simulink model "HW_StateFeedback"  (R2026a)
settings: Solver=ode1  StopTime=30  FixedStep=0.002
undefined symbols (not defined in the file): HIL, K_aug_hw, K_E_SW, K_ec, K_gs, V_sat
libraries: quarc_library x4, seesaw_hw_lib x2
settings Model: Creator=Karim Negm  LastModifiedBy=Karim Negm

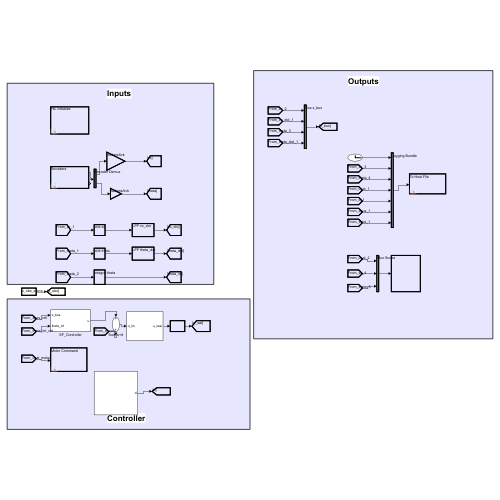
[thumbnail: Simulink's stored preview of the top-level diagram]
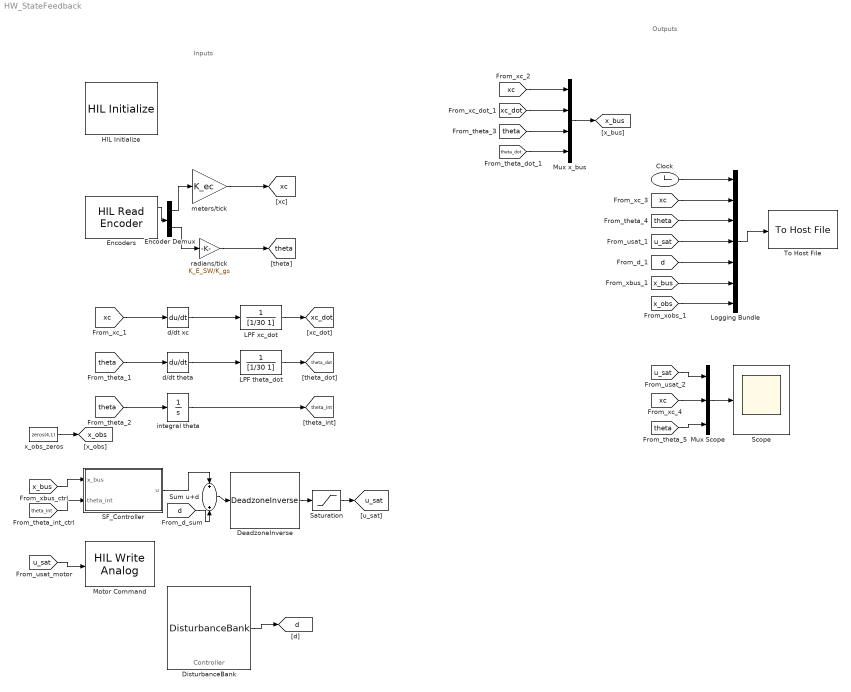
== system HW_StateFeedback ==
  note: Inputs
  note: Controller
  note: Outputs
  Clock : Clock
  DeadzoneInverse : seesaw_hw_lib/DeadzoneInverse  SystemSampleTime=-1  VariantActivationTime=update diagram  EmptyChoice=off  PassThrough=off  PassThroughVariantControl=(default)  EmptyChoiceVariantControl=(default)  AllowFlexibleInterface=on  Latency=0  AutoFrameSizeCalculation=off
  DisturbanceBank : seesaw_hw_lib/DisturbanceBank  SystemSampleTime=-1  VariantActivationTime=update diagram  EmptyChoice=off  PassThrough=off  PassThroughVariantControl=(default)  EmptyChoiceVariantControl=(default)  AllowFlexibleInterface=on  Latency=0  AutoFrameSizeCalculation=off
  Encoder Demux : Demux  Outputs=2
  Encoders : quarc_library/Data Acquisition/Generic/Immediate I//O/HIL Read Encoder  object_name=HIL-1  channels=[0:1]  sample_time=qc_get_step_size  active=on  vector_output=off  data_type_mode=Inherit via back propagation  data_type=double
  HIL Initialize : quarc_library/Data Acquisition/Generic/Configuration/HIL Initialize  object_name=HIL-1  board_type=q2_usb  board_number=0  board_options=d0=digital;d1=digital;led=auto;update_rate=normal  exclusive=off  active=off  hardware_clocks=[0:2]  clock_modes=[]  initial_clock_frequencies=[]  set_clock_params_at_start=off  set_clock_params_at_switch_in=off  set_clock_frequencies_at_start=off  set_clock_frequencies_at_switch_in=off  analog_input_channels=[0:1]  analog_input_configurations=[]  analog_input_maximums=10  analog_input_minimums=-10  set_analog_input_params_at_start=on  set_analog_input_params_at_switch_in=off  analog_output_channels=[0:1]  analog_output_maximums=10  analog_output_minimums=-10  initial_analog_outputs=[0]  final_analog_outputs=[0]  watchdog_analog_outputs=0  set_analog_output_params_at_start=on  set_analog_output_params_at_switch_in=off  set_analog_outputs_at_start=on  set_analog_outputs_at_switch_in=off  set_analog_outputs_at_terminate=on  set_analog_outputs_at_switch_out=off  set_analog_outputs_on_watchdog=off  digital_input_channels=[]  digital_output_channels=[0:7]  digital_output_configuration=[]  initial_digital_outputs=[0]  final_digital_outputs=[0]  watchdog_digital_outputs=[0]  set_digital_output_params_at_start=off  set_digital_output_params_at_switch_in=off  set_digital_outputs_at_start=on  set_digital_outputs_at_switch_in=off  set_digital_outputs_at_terminate=on  set_digital_outputs_at_switch_out=off  set_digital_outputs_on_watchdog=off  encoder_channels=[0:1]  quadrature=[4]  encoder_filter_frequency=[]  initial_encoder_counts=[0]  set_encoder_params_at_start=on  set_encoder_params_at_switch_in=off  set_encoder_counts_at_start=on  set_encoder_counts_at_switch_in=off  pwm_channels=[]  pwm_modes=[0]  pwm_frequency=1/0.020  pwm_configuration=[]  pwm_alignment=[]  pwm_polarity=[]  pwm_leading_deadband=[]  pwm_trailing_deadband=[]  initial_pwm_outputs=[0]  final_pwm_outputs=[0]  watchdog_pwm_outputs=[0]  set_pwm_params_at_start=on  set_pwm_params_at_switch_in=off  set_pwm_outputs_at_start=on  set_pwm_outputs_at_switch_in=off  set_pwm_outputs_at_terminate=on  set_pwm_outputs_at_switch_out=off  set_pwm_outputs_on_watchdog=off  other_output_channels=[]  initial_other_outputs=[]  final_other_outputs=[]  watchdog_other_outputs=[]  set_other_outputs_at_start=off  set_other_outputs_at_switch_in=off  set_other_outputs_at_terminate=off  set_other_outputs_at_switch_out=off  set_other_outputs_on_watchdog=off
  LPF theta_dot : TransferFcn  Denominator=[1/30 1]
  LPF xc_dot : TransferFcn  Denominator=[1/30 1]
  Logging Bundle : Mux  Inputs=7
  Motor Command : quarc_library/Data Acquisition/Generic/Immediate I//O/HIL Write Analog  object_name=HIL-1  channels=0  sample_time=-1  active=off  vector_input=off
  Mux Scope : Mux  Inputs=3
  Mux x_bus : Mux
  SF_Controller : Subsystem
  Saturation : Saturate  UpperLimit=V_sat  LowerLimit=-V_sat
  Scope : Scope
  Sum u+d : Sum
  To Host File : quarc_library/Sinks/To Host/To Host File  source=Specify via dialog (do not evaluate)  file_name=data_%{date}_%{time}.mat  variable_name=data  decimation=1  sample_time=-1  file_format=MAT-file v.4  options=No header or footer  append=off  final_file_name=data_05-May-2026_17-28-00.mat  encoding=Default  bitrate=0
  d/dt theta : Derivative
  d/dt xc : Derivative
  integral theta : Integrator
  meters/tick : Gain  Gain=K_ec
  radians/tick : Gain  Gain=K_E_SW/K_gs
  x_obs_zeros : Constant  Value=zeros(4,1)
  tag scope: d=global, theta=global, theta_dot=global, theta_int=global, u_sat=global, x_bus=global, x_obs=global, xc=global, xc_dot=global
  wires:
  Encoders/1 -> Encoder Demux/1
  Encoder Demux/1 -> meters/tick/1
  Encoder Demux/2 -> radians/tick/1
  meters/tick/1 -> [xc]
  radians/tick/1 -> [theta]
  [xc] -> d/dt xc/1
  d/dt xc/1 -> LPF xc_dot/1
  LPF xc_dot/1 -> [xc_dot]
  [theta] -> d/dt theta/1
  d/dt theta/1 -> LPF theta_dot/1
  LPF theta_dot/1 -> [theta_dot]
  [theta] -> integral theta/1
  integral theta/1 -> [theta_int]
  [xc] -> Mux x_bus/1
  [xc_dot] -> Mux x_bus/2
  [theta] -> Mux x_bus/3
  [theta_dot] -> Mux x_bus/4
  Mux x_bus/1 -> [x_bus]
  Clock/1 -> Logging Bundle/1
  [xc] -> Logging Bundle/2
  [theta] -> Logging Bundle/3
  [u_sat] -> Logging Bundle/4
  [d] -> Logging Bundle/5
  [x_bus] -> Logging Bundle/6
  [x_obs] -> Logging Bundle/7
  Logging Bundle/1 -> To Host File/1
  [u_sat] -> Mux Scope/1
  [xc] -> Mux Scope/2
  [theta] -> Mux Scope/3
  Mux Scope/1 -> Scope/1
  [d] -> Sum u+d/2
  Sum u+d/1 -> DeadzoneInverse/1
  DeadzoneInverse/1 -> Saturation/1
  Saturation/1 -> [u_sat]
  [u_sat] -> Motor Command/1
  DisturbanceBank/1 -> [d]
  x_obs_zeros/1 -> [x_obs]
  [x_bus] -> SF_Controller/1(x_bus)
  [theta_int] -> SF_Controller/2(theta_int)
  SF_Controller/1(u) -> Sum u+d/1

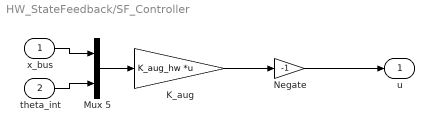
== system HW_StateFeedback/SF_Controller ==
  x_bus : Inport
  theta_int : Inport  Port=2
  K_aug : Gain  Gain=K_aug_hw  Multiplication=Matrix(K*u)
  Mux 5 : Mux  Inputs=[4 1]
  Negate : Gain  Gain=-1
  u : Outport
  wires:
  x_bus/1 -> Mux 5/1
  theta_int/1 -> Mux 5/2
  Mux 5/1 -> K_aug/1
  K_aug/1 -> Negate/1
  Negate/1 -> u/1
